simulink model "simulate_3pools"  (R2019b)
settings: Solver=FixedStepDiscrete  StartTime=0.0  StopTime=60*30  FixedStep=1  RelTol=1e-3
values from neighbouring files (symbols this model uses):
  comb_contr = ss(Ac, Bc, Cc, Dc, h)    [cantoni_LMI.m]
  comb_plant_disc = c2d(comb_plant_cont,h,'zoh')    [cantoni_LMI.m]
  ddelay = [4 2 4 4 6]    [distributed_workspace.mat]
  Pd0 = c2d(P0, h, 'zoh')    [model_hil.m]
undefined symbols (not defined in the file or in its folder): comb_K_disc, comb_Pool_disc, Pd, Wd
settings Model: Creator=Jacob  LastModifiedBy=bas
settings DataIOCC: ReturnWorkspaceOutputs=off
settings SFSimCC: CustomCodeUndefinedFunction=UseInterfaceOnly

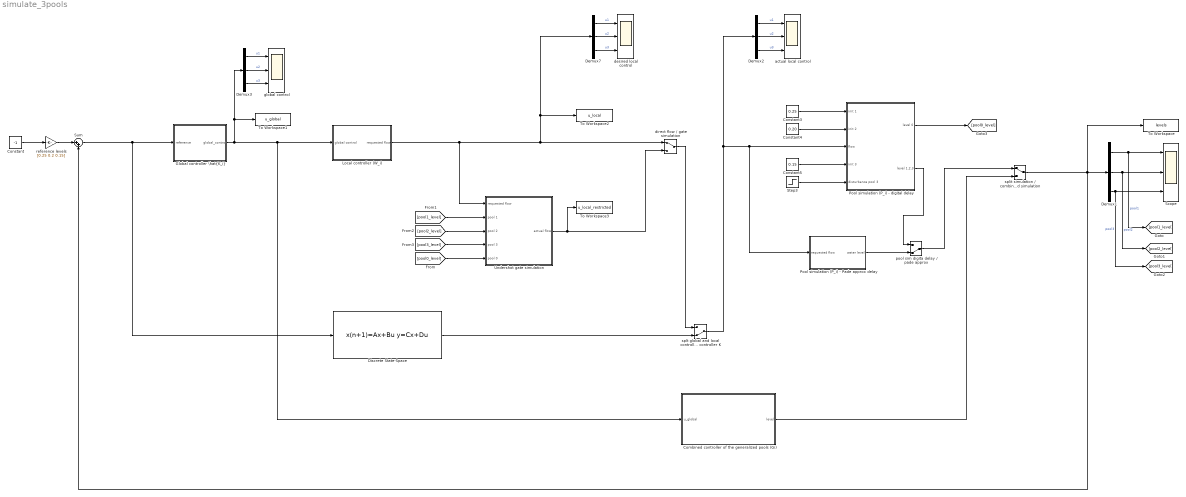
== system simulate_3pools ==
  Combined controller of the generalized pools (Gi) : Subsystem
  Constant : Constant  Value=-1
  Constant3 : Constant  Value=0.25  SampleTime=-1
  Constant4 : Constant  Value=0.20
  Constant5 : Constant  Value=0.15
  Demux{1..3,7} (4 alike) : Demux  Outputs=3
  Discrete State-Space : DiscreteStateSpace  A=comb_K_disc.A  B=comb_K_disc.B  C=comb_K_disc.C  D=comb_K_disc.D  SampleTime=-1
  "Global controller \\hat{K_i}" : Subsystem
  Local controller (W_i) : Subsystem
  Pool simulation (P_i) - Pade approx delay : Subsystem
  Pool simulation (P_i) - digital delay : Subsystem
  Scope : Scope  NumInputPorts=3
  Step3 : Step  Time=100  After=-0.015  SampleTime=0
  Sum : Sum  Inputs=|++
  To Workspace : ToWorkspace  VariableName=levels  SaveFormat=Timeseries  SampleTime=-1
  To Workspace1 : ToWorkspace  VariableName=u_global  SaveFormat=Timeseries  SampleTime=-1
  To Workspace2 : ToWorkspace  VariableName=u_local  SaveFormat=Timeseries  SampleTime=-1
  To Workspace3 : ToWorkspace  VariableName=u_local_restricted  SaveFormat=Timeseries  SampleTime=-1
  Undershot gate simulation : Subsystem
  actual local control : Scope  NumInputPorts=3
  desired local control : Scope  NumInputPorts=3
  direct flow / gate simulation : ManualSwitch
  global control : Scope  NumInputPorts=3
  pool sim digita delay / pade approx : ManualSwitch  CurrentSetting=0
  reference levels : Gain  Gain=[0.25 0.2 0.15]
  split simulation / combined simulation : ManualSwitch
  splt global and local controllers / combined controller K : ManualSwitch  CurrentSetting=0
  wires:
  Constant/1 -> reference levels/1
  reference levels/1 -> Sum/1
  split simulation / combined simulation/1 -> To Workspace/1, Demux1/1, Sum/2
  Demux1/1 -> Scope/1, [pool1_level]  "pool1"
  Demux1/2 -> [pool2_level], Scope/2  "pool2"
  Demux1/3 -> [pool3_level], Scope/3  "pool3"
  Demux3/3 -> global control/3  "u3"
  Demux3/2 -> global control/2  "u2"
  Demux3/1 -> global control/1  "u1"
  "Global controller \\hat{K_i}"/1(global_control) -> To Workspace1/1, Demux3/1, Combined controller of the generalized pools (Gi)/1(u_global), Local controller (W_i)/1(global control)
  Sum/1 -> Discrete State-Space/1, "Global controller \\hat{K_i}"/1(reference)
  Demux2/3 -> actual local control/3  "u3"
  Demux2/1 -> actual local control/1  "u1"
  Demux2/2 -> actual local control/2  "u2"
  Demux7/3 -> desired local control/3  "u3"
  Demux7/2 -> desired local control/2  "u2"
  Demux7/1 -> desired local control/1  "u1"
  Local controller (W_i)/1(requested flow) -> Undershot gate simulation/1(requested flow), direct flow / gate simulation/1, Demux7/1, To Workspace2/1
  Undershot gate simulation/1(actual flow) -> direct flow / gate simulation/2, To Workspace3/1
  [pool1_level] -> Undershot gate simulation/2(pool 1)
  [pool2_level] -> Undershot gate simulation/3(pool 2)
  [pool3_level] -> Undershot gate simulation/4(pool 3)
  [pool0_level] -> Undershot gate simulation/5(pool 0)
  Constant3/1 -> Pool simulation (P_i) - digital delay/1(init 1)
  Constant4/1 -> Pool simulation (P_i) - digital delay/2(init 2)
  Constant5/1 -> Pool simulation (P_i) - digital delay/4(init 3)
  Step3/1 -> Pool simulation (P_i) - digital delay/5(disturbance pool 3)
  Pool simulation (P_i) - digital delay/1(level 0) -> [pool0_level]
  pool sim digita delay / pade approx/1 -> split simulation / combined simulation/1
  Pool simulation (P_i) - digital delay/2(level 1,2,3) -> pool sim digita delay / pade approx/1
  splt global and local controllers / combined controller K/1 -> Demux2/1, Pool simulation (P_i) - Pade approx delay/1(requested flow), Pool simulation (P_i) - digital delay/3(flow)
  Pool simulation (P_i) - Pade approx delay/1(water level) -> pool sim digita delay / pade approx/2
  Combined controller of the generalized pools (Gi)/1(level) -> split simulation / combined simulation/2
  direct flow / gate simulation/1 -> splt global and local controllers / combined controller K/1
  Discrete State-Space/1 -> splt global and local controllers / combined controller K/2

== system simulate_3pools/Combined controller of the generalized pools (Gi) ==
  u_global : Inport
  Combined controller of the generalized pools (Gi) : DiscreteStateSpace  A=comb_plant_disc.A  B=comb_plant_disc.B  C=comb_plant_disc.C  D=comb_plant_disc.D  SampleTime=-1
  Combined controller of the generalized pools (Gi) with disturbance (outtake pool 3) : Subsystem
  no disturbance / disturbance (combined local + pools) : ManualSwitch  CurrentSetting=0
  level : Outport
  wires:
  no disturbance / disturbance (combined local + pools)/1 -> level/1
  Combined controller of the generalized pools (Gi) with disturbance (outtake pool 3)/1(water_level) -> no disturbance / disturbance (combined local + pools)/2
  u_global/1 -> Combined controller of the generalized pools (Gi) with disturbance (outtake pool 3)/1(u_global), Combined controller of the generalized pools (Gi)/1
  Combined controller of the generalized pools (Gi)/1 -> no disturbance / disturbance (combined local + pools)/1

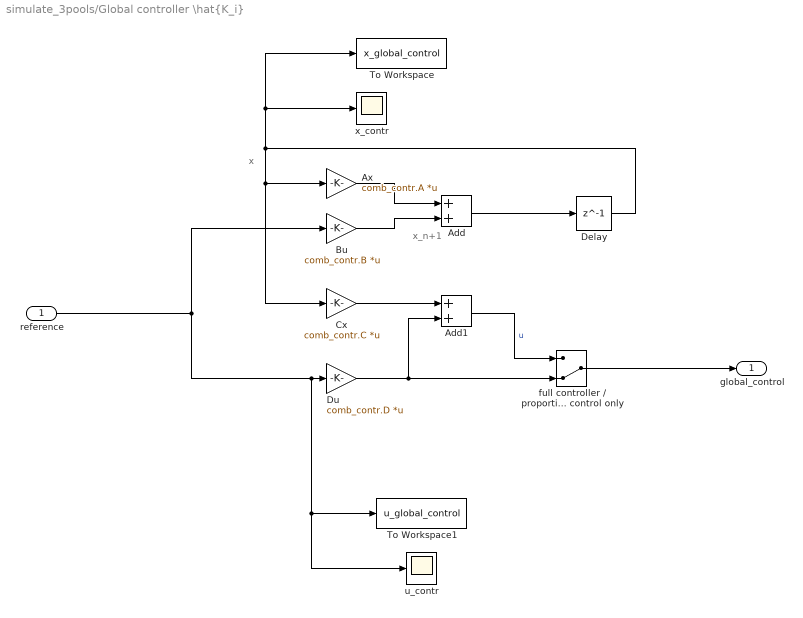
== system simulate_3pools/Global controller \hat{K_i} ==
  note: x
  note: x_n+1
  reference : Inport
  Add : Sum
  Add1 : Sum
  Ax : Gain  Gain=comb_contr.A  Multiplication=Matrix(K*u)
  Bu : Gain  Gain=comb_contr.B  Multiplication=Matrix(K*u)
  Cx : Gain  Gain=comb_contr.C  Multiplication=Matrix(K*u)
  Delay : Delay  DelayLength=1  InitialCondition=[0;0;0;0;0;0;0;0;0;0;0;0;0;0;0]
  Du : Gain  Gain=comb_contr.D  Multiplication=Matrix(K*u)
  To Workspace : ToWorkspace  VariableName=x_global_control  SaveFormat=Timeseries  SampleTime=-1
  To Workspace1 : ToWorkspace  VariableName=u_global_control  SaveFormat=Timeseries  SampleTime=-1
  full controller / proportional control only : ManualSwitch  CurrentSetting=0
  u_contr : Scope
  x_contr : Scope
  global_control : Outport
  wires:
  Bu/1 -> Add/2
  Cx/1 -> Add1/1
  Add/1 -> Delay/1
  Add1/1 -> full controller / proportional control only/1  "u"
  Ax/1 -> Add/1
  Du/1 -> Add1/2, full controller / proportional control only/2
  full controller / proportional control only/1 -> global_control/1
  reference/1 -> To Workspace1/1, u_contr/1, Du/1, Bu/1
  Delay/1 -> To Workspace/1, x_contr/1, Cx/1, Ax/1

== system simulate_3pools/Local controller (W_i) ==
  global control : Inport
  firefly implementation / transfer functions : ManualSwitch  CurrentSetting=0
  local controller implementations : Subsystem
  local controller transfer functions : Subsystem
  requested flow : Outport
  wires:
  firefly implementation / transfer functions/1 -> requested flow/1  "requested flow"
  local controller transfer functions/1(local_control) -> firefly implementation / transfer functions/2
  global control/1 -> local controller transfer functions/1(global_control_in), local controller implementations/1(global_control_in)
  local controller implementations/1(local_control) -> firefly implementation / transfer functions/1

== system simulate_3pools/Pool simulation (P_i) - Pade approx delay ==
  requested flow : Inport
  Combined pools with Pade delay and disturbance : Subsystem
  Discrete State-Space : DiscreteStateSpace  A=comb_Pool_disc.A  B=comb_Pool_disc.B  C=comb_Pool_disc.C  D=comb_Pool_disc.D  SampleTime=-1
  no disturbance / disturbance (pools) : ManualSwitch  CurrentSetting=0
  water level : Outport
  wires:
  Discrete State-Space/1 -> no disturbance / disturbance (pools)/1
  no disturbance / disturbance (pools)/1 -> water level/1
  requested flow/1 -> Combined pools with Pade delay and disturbance/1(requested flow), Discrete State-Space/1
  Combined pools with Pade delay and disturbance/1(level) -> no disturbance / disturbance (pools)/2

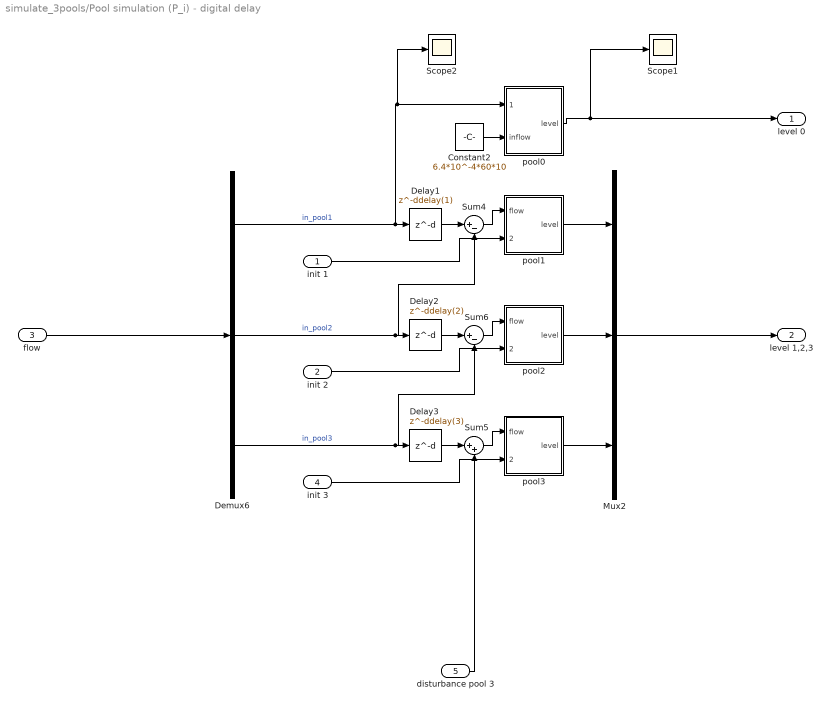
== system simulate_3pools/Pool simulation (P_i) - digital delay ==
  init 1 : Inport
  init 2 : Inport  Port=2
  flow : Inport  Port=3
  init 3 : Inport  Port=4
  disturbance pool 3 : Inport  Port=5
  Constant2 : Constant  Value=6.4*10^-4*60*10
  Delay1 : Delay  DelayLength=ddelay(1)
  Delay2 : Delay  DelayLength=ddelay(2)
  Delay3 : Delay  DelayLength=ddelay(3)
  Demux6 : Demux  Outputs=3
  Mux2 : Mux  Inputs=3
  Scope1 : Scope
  Scope2 : Scope
  Sum4 : Sum  Inputs=|+-
  Sum5 : Sum  Inputs=|++
  Sum6 : Sum  Inputs=|+-
  pool0 : Subsystem
  pool1 : Subsystem
  pool2 : Subsystem
  pool3 : Subsystem
  level 0 : Outport
  level 1,2,3 : Outport  Port=2
  wires:
  init 1/1 -> pool1/2("initial_level ")
  init 3/1 -> pool3/2(initial_level)
  Sum6/1 -> pool2/1(flow)
  pool2/1(level) -> Mux2/2
  Delay3/1 -> Sum5/1
  disturbance pool 3/1 -> Sum5/2
  Demux6/3 -> Sum6/2, Delay3/1  "in_pool3"
  pool3/1(level) -> Mux2/3
  pool1/1(level) -> Mux2/1
  Constant2/1 -> pool0/2(inflow)
  pool0/1(level) -> level 0/1, Scope1/1
  Sum4/1 -> pool1/1(flow)
  Mux2/1 -> level 1,2,3/1
  Sum5/1 -> pool3/1(flow)
  Demux6/2 -> Sum4/2, Delay2/1  "in_pool2"
  init 2/1 -> pool2/2(initial_level)
  Delay2/1 -> Sum6/1
  Delay1/1 -> Sum4/1
  flow/1 -> Demux6/1
  Demux6/1 -> Scope2/1, pool0/1(outflow), Delay1/1  "in_pool1"

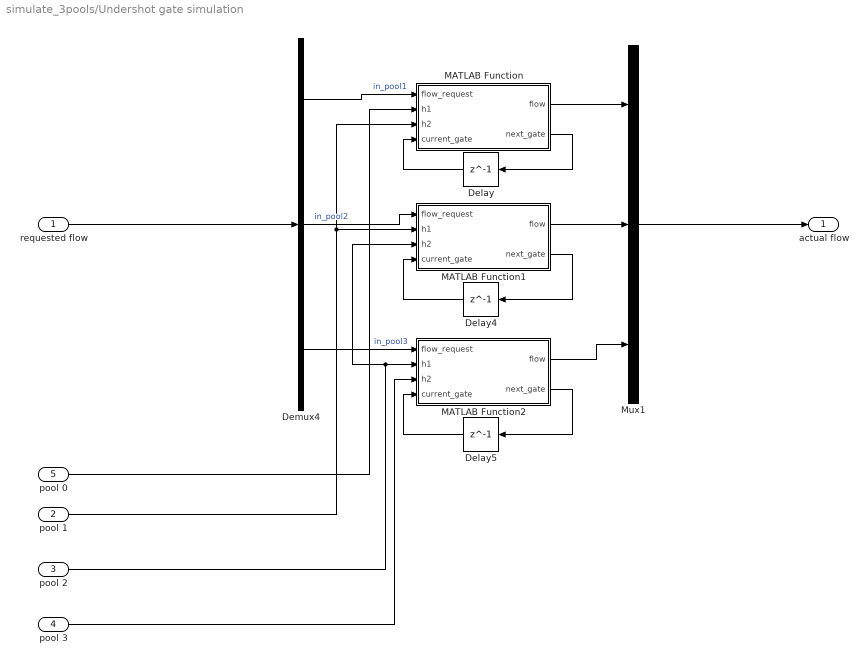
== system simulate_3pools/Undershot gate simulation ==
  requested flow : Inport
  pool 1 : Inport  Port=2
  pool 2 : Inport  Port=3
  pool 3 : Inport  Port=4
  pool 0 : Inport  Port=5
  Delay : Delay  DelayLength=1
  Delay4 : Delay  DelayLength=1
  Delay5 : Delay  DelayLength=1
  Demux4 : Demux  Outputs=3
  MATLAB Function : MATLAB Function  TreatAsAtomicUnit=on
  MATLAB Function1 : MATLAB Function  TreatAsAtomicUnit=on
  MATLAB Function2 : MATLAB Function  TreatAsAtomicUnit=on
  Mux1 : Mux  Inputs=3
  actual flow : Outport
  wires:
  requested flow/1 -> Demux4/1
  Demux4/1 -> MATLAB Function/1(flow_request)  "in_pool1"
  pool 0/1 -> MATLAB Function/2(h1)
  MATLAB Function2/1(flow) -> Mux1/3
  Demux4/3 -> MATLAB Function2/1(flow_request)  "in_pool3"
  MATLAB Function1/2(next_gate) -> Delay4/1
  pool 3/1 -> MATLAB Function2/3(h2)
  MATLAB Function2/2(next_gate) -> Delay5/1
  Demux4/2 -> MATLAB Function1/1(flow_request)  "in_pool2"
  MATLAB Function1/1(flow) -> Mux1/2
  Mux1/1 -> actual flow/1
  Delay/1 -> MATLAB Function/4(current_gate)
  pool 1/1 -> MATLAB Function1/2(h1), MATLAB Function/3(h2)
  MATLAB Function/2(next_gate) -> Delay/1
  Delay5/1 -> MATLAB Function2/4(current_gate)
  pool 2/1 -> MATLAB Function1/3(h2), MATLAB Function2/2(h1)
  Delay4/1 -> MATLAB Function1/4(current_gate)
  MATLAB Function/1(flow) -> Mux1/1

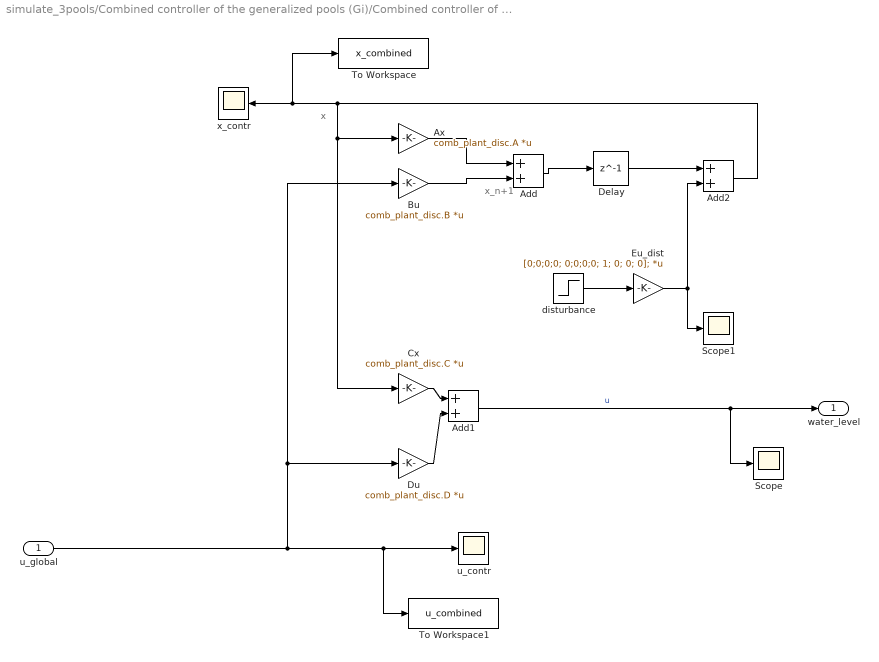
== system simulate_3pools/Combined controller of the generalized pools (Gi)/Combined controller of the generalized pools (Gi) with disturbance (outtake pool 3) ==
  note: x
  note: x_n+1
  u_global : Inport
  Add : Sum
  Add1 : Sum
  Add2 : Sum
  Ax : Gain  Gain=comb_plant_disc.A  Multiplication=Matrix(K*u)
  Bu : Gain  Gain=comb_plant_disc.B  Multiplication=Matrix(K*u)
  Cx : Gain  Gain=comb_plant_disc.C  Multiplication=Matrix(K*u)
  Delay : Delay  DelayLength=1  InitialCondition=[0.25;0;0;0;0.20;0;0;0;0.15;0;0;0]
  Du : Gain  Gain=comb_plant_disc.D  Multiplication=Matrix(K*u)
  Eu_dist : Gain  Gain=[0;0;0;0; 0;0;0;0; 1; 0; 0; 0];  Multiplication=Matrix(K*u)
  Scope : Scope
  Scope1 : Scope
  To Workspace : ToWorkspace  VariableName=x_combined  SaveFormat=Timeseries  SampleTime=-1
  To Workspace1 : ToWorkspace  VariableName=u_combined  SaveFormat=Timeseries  SampleTime=-1
  disturbance : Step  Time=100  After=-0.015/0.2279* 1/60  SampleTime=0
  u_contr : Scope
  x_contr : Scope
  water_level : Outport
  wires:
  Bu/1 -> Add/2
  Cx/1 -> Add1/1
  Add/1 -> Delay/1
  Add1/1 -> Scope/1, water_level/1  "u"
  Ax/1 -> Add/1
  Du/1 -> Add1/2
  Add2/1 -> To Workspace/1, x_contr/1, Cx/1, Ax/1
  u_global/1 -> To Workspace1/1, u_contr/1, Du/1, Bu/1
  disturbance/1 -> Eu_dist/1
  Eu_dist/1 -> Add2/2, Scope1/1
  Delay/1 -> Add2/1

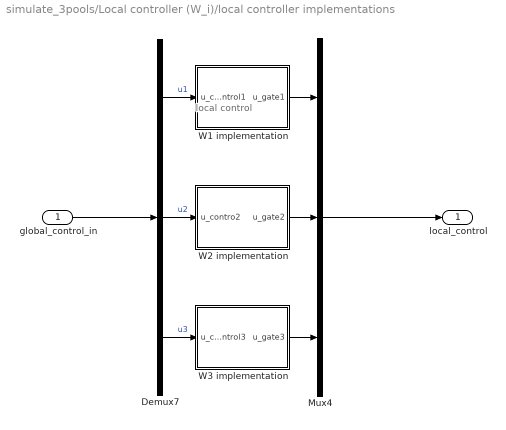
== system simulate_3pools/Local controller (W_i)/local controller implementations ==
  note: local control
  global_control_in : Inport
  Demux7 : Demux  Outputs=3
  Mux4 : Mux  Inputs=3
  W1 implementation : Subsystem
  W2 implementation : Subsystem
  W3 implementation : Subsystem
  local_control : Outport
  wires:
  Demux7/1 -> W1 implementation/1(u_control1)  "u1"
  W1 implementation/1(u_gate1) -> Mux4/1
  Demux7/3 -> W3 implementation/1(u_control3)  "u3"
  Demux7/2 -> W2 implementation/1(u_contro2)  "u2"
  global_control_in/1 -> Demux7/1
  Mux4/1 -> local_control/1
  W3 implementation/1(u_gate3) -> Mux4/3
  W2 implementation/1(u_gate2) -> Mux4/2

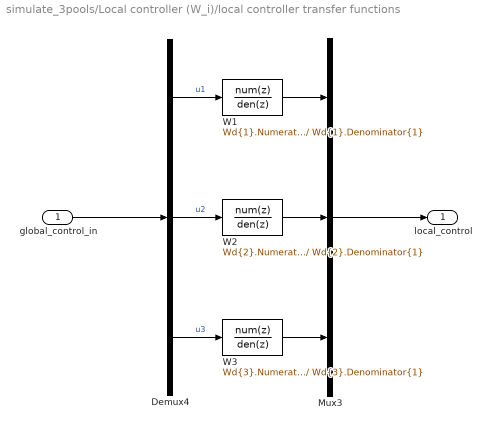
== system simulate_3pools/Local controller (W_i)/local controller transfer functions ==
  global_control_in : Inport
  Demux4 : Demux  Outputs=3
  Mux3 : Mux  Inputs=3
  W1 : DiscreteTransferFcn  Numerator=Wd{1}.Numerator{1}  Denominator=Wd{1}.Denominator{1}
  W2 : DiscreteTransferFcn  Numerator=Wd{2}.Numerator{1}  Denominator=Wd{2}.Denominator{1}
  W3 : DiscreteTransferFcn  Numerator=Wd{3}.Numerator{1}  Denominator=Wd{3}.Denominator{1}
  local_control : Outport
  wires:
  Mux3/1 -> local_control/1
  global_control_in/1 -> Demux4/1
  Demux4/3 -> W3/1  "u3"
  W3/1 -> Mux3/3
  Demux4/2 -> W2/1  "u2"
  W2/1 -> Mux3/2
  W1/1 -> Mux3/1
  Demux4/1 -> W1/1  "u1"

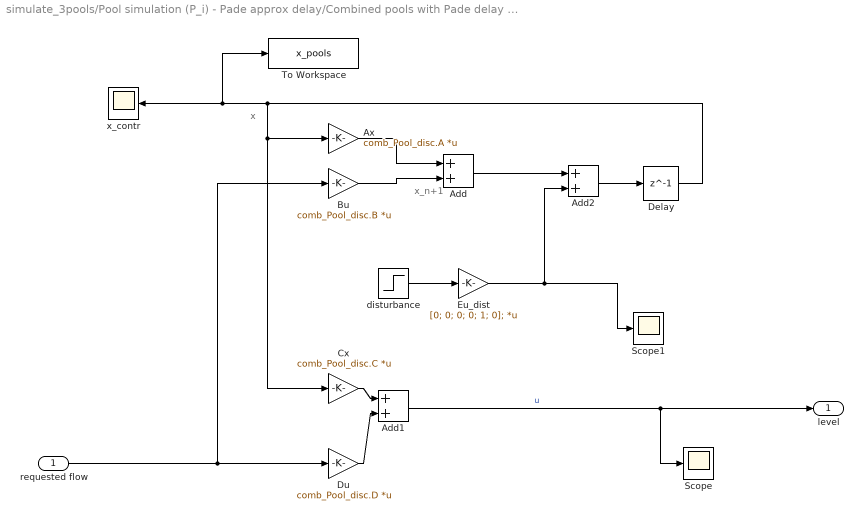
== system simulate_3pools/Pool simulation (P_i) - Pade approx delay/Combined pools with Pade delay and disturbance ==
  note: x_n+1
  note: x
  requested flow : Inport
  Add : Sum
  Add1 : Sum
  Add2 : Sum
  Ax : Gain  Gain=comb_Pool_disc.A  Multiplication=Matrix(K*u)
  Bu : Gain  Gain=comb_Pool_disc.B  Multiplication=Matrix(K*u)
  Cx : Gain  Gain=comb_Pool_disc.C  Multiplication=Matrix(K*u)
  Delay : Delay  DelayLength=1  InitialCondition=[0.25;0;0.2;0;0.15;0]
  Du : Gain  Gain=comb_Pool_disc.D  Multiplication=Matrix(K*u)
  Eu_dist : Gain  Gain=[0; 0; 0; 0; 1; 0];  Multiplication=Matrix(K*u)
  Scope : Scope
  Scope1 : Scope
  To Workspace : ToWorkspace  VariableName=x_pools  SaveFormat=Timeseries  SampleTime=-1
  disturbance : Step  Time=100  After=-0.015/0.2279* 1/60  SampleTime=0
  x_contr : Scope
  level : Outport
  wires:
  disturbance/1 -> Eu_dist/1
  Ax/1 -> Add/1
  Bu/1 -> Add/2
  Add/1 -> Add2/1
  requested flow/1 -> Bu/1, Du/1
  Add1/1 -> level/1, Scope/1  "u"
  Cx/1 -> Add1/1
  Eu_dist/1 -> Scope1/1, Add2/2
  Du/1 -> Add1/2
  Delay/1 -> To Workspace/1, x_contr/1, Cx/1, Ax/1
  Add2/1 -> Delay/1

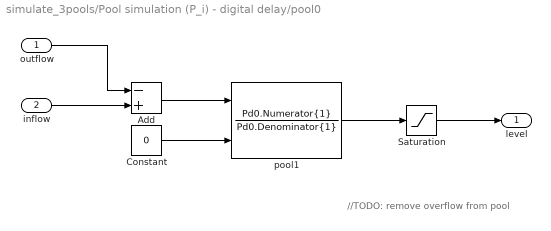
== system simulate_3pools/Pool simulation (P_i) - digital delay/pool0 ==
  note: //TODO: remove overflow from pool
  outflow : Inport
  inflow : Inport  Port=2
  Add : Sum  Inputs=-+
  Constant : Constant  Value=0
  Saturation : Saturate  UpperLimit=0.3
  pool1 : DiscreteTransferFcn  Numerator=Pd0.Numerator{1}  Denominator=Pd0.Denominator{1}  InitialStatesSource=Input port
      settings: InputPortMap=u0,p5
  level : Outport
  wires:
  pool1/1 -> Saturation/1
  outflow/1 -> Add/1
  inflow/1 -> Add/2
  Add/1 -> pool1/1
  Constant/1 -> pool1/2
  Saturation/1 -> level/1

== system simulate_3pools/Pool simulation (P_i) - digital delay/pool1 ==
  flow : Inport
  "initial_level " : Inport  Port=2
  Gain : Gain  Gain=1/Pd{1}.Numerator{1}(2)
  P1 : DiscreteTransferFcn  Numerator=Pd{1}.Numerator{1}  Denominator=Pd{1}.Denominator{1}  InitialStatesSource=Input port
      settings: InputPortMap=u0,p5
  level : Outport
  wires:
  flow/1 -> P1/1
  P1/1 -> level/1
  Gain/1 -> P1/2
  "initial_level "/1 -> Gain/1

== system simulate_3pools/Pool simulation (P_i) - digital delay/pool2 ==
  flow : Inport
  initial_level : Inport  Port=2
  Gain : Gain  Gain=1/Pd{2}.Numerator{1}(2)
  P2 : DiscreteTransferFcn  Numerator=Pd{2}.Numerator{1}  Denominator=Pd{2}.Denominator{1}  InitialStatesSource=Input port
      settings: InputPortMap=u0,p5
  level : Outport
  wires:
  flow/1 -> P2/1
  P2/1 -> level/1
  Gain/1 -> P2/2
  initial_level/1 -> Gain/1

== system simulate_3pools/Pool simulation (P_i) - digital delay/pool3 ==
  flow : Inport
  initial_level : Inport  Port=2
  Gain : Gain  Gain=1/Pd{3}.Numerator{1}(2)
  P3 : DiscreteTransferFcn  Numerator=Pd{3}.Numerator{1}  Denominator=Pd{3}.Denominator{1}  InitialStatesSource=Input port
      settings: InputPortMap=u0,p5
  level : Outport
  wires:
  P3/1 -> level/1
  flow/1 -> P3/1
  Gain/1 -> P3/2
  initial_level/1 -> Gain/1

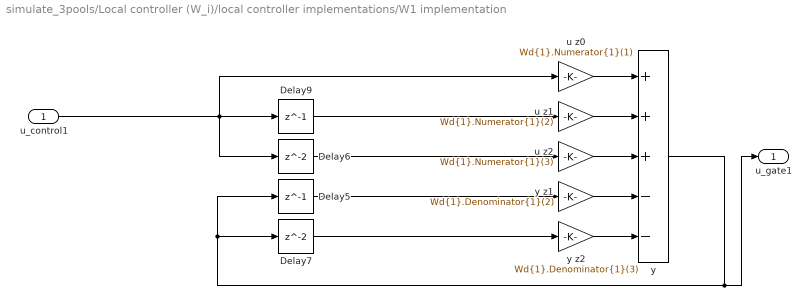
== system simulate_3pools/Local controller (W_i)/local controller implementations/W1 implementation ==
  u_control1 : Inport
  Delay5 : Delay  DelayLength=1
  Delay6 : Delay
  Delay7 : Delay
  Delay9 : Delay  DelayLength=1
  u z0 : Gain  Gain=Wd{1}.Numerator{1}(1)
  u z1 : Gain  Gain=Wd{1}.Numerator{1}(2)
  u z2 : Gain  Gain=Wd{1}.Numerator{1}(3)
  y : Sum  Inputs=+++--
  y z1 : Gain  Gain=Wd{1}.Denominator{1}(2)
  y z2 : Gain  Gain=Wd{1}.Denominator{1}(3)
  u_gate1 : Outport
  wires:
  y z2/1 -> y/5
  Delay6/1 -> u z2/1
  y z1/1 -> y/4
  Delay7/1 -> y z2/1
  u z1/1 -> y/2
  u z2/1 -> y/3
  Delay5/1 -> y z1/1
  u_control1/1 -> Delay6/1, u z0/1, Delay9/1
  u z0/1 -> y/1
  Delay9/1 -> u z1/1
  y/1 -> u_gate1/1, Delay5/1, Delay7/1

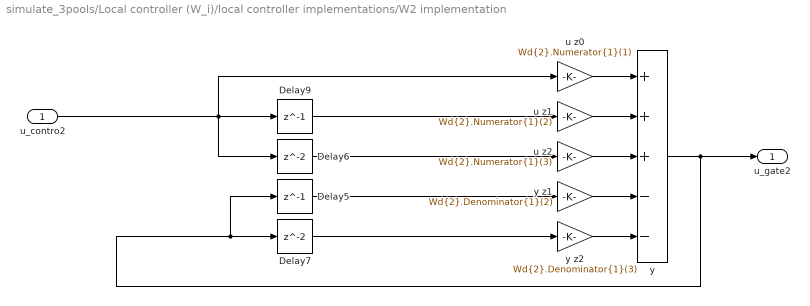
== system simulate_3pools/Local controller (W_i)/local controller implementations/W2 implementation ==
  u_contro2 : Inport
  Delay5 : Delay  DelayLength=1
  Delay6 : Delay
  Delay7 : Delay
  Delay9 : Delay  DelayLength=1
  u z0 : Gain  Gain=Wd{2}.Numerator{1}(1)
  u z1 : Gain  Gain=Wd{2}.Numerator{1}(2)
  u z2 : Gain  Gain=Wd{2}.Numerator{1}(3)
  y : Sum  Inputs=+++--
  y z1 : Gain  Gain=Wd{2}.Denominator{1}(2)
  y z2 : Gain  Gain=Wd{2}.Denominator{1}(3)
  u_gate2 : Outport
  wires:
  y z2/1 -> y/5
  Delay6/1 -> u z2/1
  y z1/1 -> y/4
  Delay7/1 -> y z2/1
  u z1/1 -> y/2
  u z2/1 -> y/3
  Delay5/1 -> y z1/1
  u_contro2/1 -> Delay6/1, u z0/1, Delay9/1
  u z0/1 -> y/1
  Delay9/1 -> u z1/1
  y/1 -> Delay5/1, Delay7/1, u_gate2/1

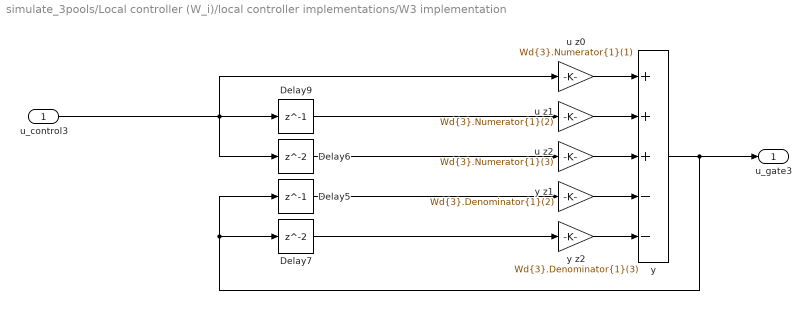
== system simulate_3pools/Local controller (W_i)/local controller implementations/W3 implementation ==
  u_control3 : Inport
  Delay5 : Delay  DelayLength=1
  Delay6 : Delay
  Delay7 : Delay
  Delay9 : Delay  DelayLength=1
  u z0 : Gain  Gain=Wd{3}.Numerator{1}(1)
  u z1 : Gain  Gain=Wd{3}.Numerator{1}(2)
  u z2 : Gain  Gain=Wd{3}.Numerator{1}(3)
  y : Sum  Inputs=+++--
  y z1 : Gain  Gain=Wd{3}.Denominator{1}(2)
  y z2 : Gain  Gain=Wd{3}.Denominator{1}(3)
  u_gate3 : Outport
  wires:
  y z2/1 -> y/5
  Delay6/1 -> u z2/1
  y z1/1 -> y/4
  Delay7/1 -> y z2/1
  u z1/1 -> y/2
  u z2/1 -> y/3
  Delay5/1 -> y z1/1
  u_control3/1 -> Delay6/1, u z0/1, Delay9/1
  u z0/1 -> y/1
  Delay9/1 -> u z1/1
  y/1 -> Delay5/1, Delay7/1, u_gate3/1

== matlab function simulate_3pools/Undershot gate simulation/MATLAB Function1 ==
  data: flow_request input; flow output; h1 input; h2 input; current_gate input; next_gate output
function [flow, next_gate] = fcn(flow_request, h1, h2, current_gate)

[flow, next_gate] = gate_simulation(flow_request, h1, h2, current_gate);

== matlab function simulate_3pools/Undershot gate simulation/MATLAB Function ==
  data: flow_request input; flow output; h1 input; h2 input; current_gate input; next_gate output
function [flow, next_gate] = fcn(flow_request, h1, h2, current_gate)

[flow, next_gate] = gate_simulation(flow_request, h1, h2, current_gate);

== matlab function simulate_3pools/Undershot gate simulation/MATLAB Function2 ==
  data: flow_request input; flow output; h1 input; h2 input; current_gate input; next_gate output
function [flow, next_gate] = fcn(flow_request, h1, h2, current_gate)

[flow, next_gate] = gate_simulation(flow_request, h1, h2, current_gate);
